simulink model "GuiamentoControle"  (R2024a)
settings: Solver=FixedStepAuto  StartTime=0.0  StopTime=C.Tfim  FixedStep=0.01  MaxStep=0.001  RelTol=1e-3
values from neighbouring files (symbols this model uses):
  C = CondLanc6DOF    [RunGuiamentoDiag.m]    (also in RunGuiamentoFull.m; RunGuiamentoPlots.m; VooUnico6DOF.m)
  cte_grav = 9.8    [CondLanc6DOF.m]    (also in DadosControle.m; DadosMissil.m; Envelope6DOF.m; RunGuiamentoDiag.m)
  D = DadosControle(D)    [Envelope6DOF.m]    (also in ProjContAlt.m = DadosCGInercia(D); ProjRLocus.m = DadosCGInercia(D); RunGuiamentoDiag.m; RunGuiamentoFull.m)
  R2D = 180/pi    (= 57.2957795131)    [DadosControle.m]    (also in Envelope6DOF.m; RunGuiamentoDiag.m; RunGuiamentoFull.m; RunGuiamentoPlots.m)
  T_acel_k_ext = [0.103333333333 0.121666666667 0.126666666667 0.116666666667 0.143333333333 0.196666666667 0.103333333333 0.121666666667 0.126666666667 0.116666666667 0.143333333333 0.193333333333 ... (36 elements, 6x2x3)]    [autopiloto.mat]    (also in autopiloto_antiship.mat = [0.00333333333333 0.00333333333333 0.00333333333333 0.006666)
  T_acel_k_int = [0.788 0.796 0.789 0.757 0.742 0.695 0.792 0.8 0.793 0.761 0.746 0.699 ... (36 elements, 6x2x3)]    [autopiloto.mat]    (also in autopiloto_antiship.mat = [0.786666666667 1.01333333333 1.14666666667 1.18666666667 1.)
  T_at_k_ext = zeros(length(x_CG),length(altitude),length(Mach))    [ProjRLocus.m]    (also in autopiloto.mat = [5.525 6.1 7.1625 8.4375 9.9 12.1875 5.4875 6.0625 7.1125 8.; autopiloto_antiship.mat = [9.33333333333 13.3333333333 18.6666666667 24 34.6666666667 )
  T_at_k_int = zeros(length(x_CG),length(altitude),length(Mach))    [ProjRLocus.m]    (also in autopiloto.mat = [0.788 0.796 0.789 0.757 0.742 0.695 0.792 0.8 0.793 0.761 0; autopiloto_antiship.mat = [0.786666666667 1.01333333333 1.14666666667 1.18666666667 1.)
  vet_altitude = altitude    [ProjRLocus.m]    (also in autopiloto.mat = [10 100]; autopiloto_antiship.mat = [10 100])
  vet_Mach = Mach    [ProjRLocus.m]    (also in autopiloto.mat = [0.6 0.75 0.9]; autopiloto_antiship.mat = [0.6 0.75 0.9 1])
  vet_x_CG = x_CG    [ProjRLocus.m]    (also in autopiloto.mat = [-2.56109748385 -2.4846531203 -2.35211691443 -2.20935548439 ; autopiloto_antiship.mat = [-2.98430726841 -2.86504003942 -2.66873079492 -2.47886843287)
undefined symbols (not defined in the file or in its folder): dados, M_CD, M_CM, M_CMQ, M_CN, Newton, Raphson
libraries: simulink x14, aerolibasang x9, shared6dof x5, sharedutil x3, aerolibatmos2 x1, dspmtrx3 x1
(part 1 of 2)
settings Model: Creator=carlberto-old  LastModifiedBy=mathe
settings SolverCC: AlgebraicLoopSolver=LineSearch
settings DataIOCC: ReturnWorkspaceOutputs=off
settings DebuggingCC: UnconnectedInputMsg=warning  UnconnectedOutputMsg=warning  UnconnectedLineMsg=warning  ArithmeticOperatorsInVariantConditions=warning
settings ModelReferenceCC: EnableRefExpFcnMdlSchedulingChecks=on
settings SFSimCC: SimUseLocalCustomCode=off  CustomCodeUndefinedFunction=UseInterfaceOnly
settings RTWCC: RTWUseLocalCustomCode=off  GPUComputeCapability=3.5

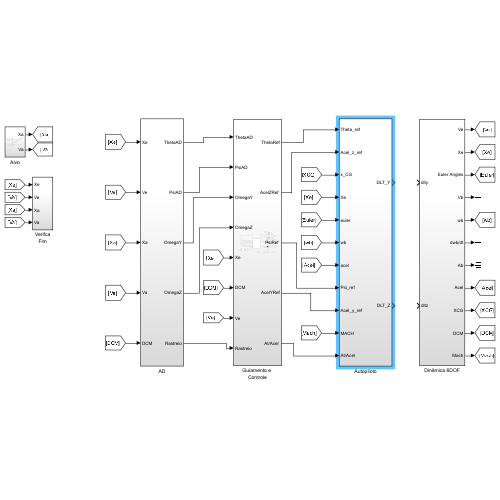
[thumbnail: Simulink's stored preview of the top-level diagram]
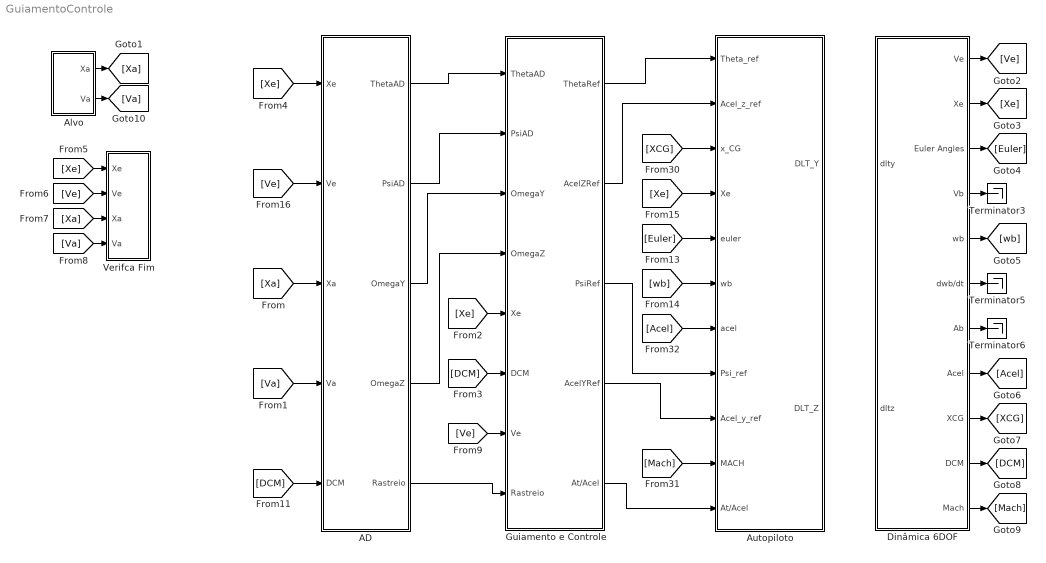
== system GuiamentoControle ==
  "AD " : Subsystem
  Alvo : Subsystem
  Autopiloto : Subsystem
  Dinâmica 6DOF : Subsystem
  Guiamento e Controle : Subsystem
  Terminator3 : Terminator
  Terminator5 : Terminator
  Terminator6 : Terminator
  Verifca Fim : Subsystem
  wires:
  Dinâmica 6DOF/2(Xe) -> [Xe]
  Dinâmica 6DOF/3(Euler Angles) -> [Euler]
  Dinâmica 6DOF/5(wb) -> [wb]
  Dinâmica 6DOF/1(Ve) -> [Ve]
  Dinâmica 6DOF/7(Ab) -> Terminator6/1
  Dinâmica 6DOF/6(dwb/dt) -> Terminator5/1
  Dinâmica 6DOF/4(Vb) -> Terminator3/1
  Dinâmica 6DOF/10(DCM) -> [DCM]
  Dinâmica 6DOF/9(XCG) -> [XCG]
  Dinâmica 6DOF/8(Acel) -> [Acel]
  Dinâmica 6DOF/11(Mach) -> [Mach]
  [XCG] -> Autopiloto/3(x_CG)
  [wb] -> Autopiloto/6(wb)
  [Euler] -> Autopiloto/5(euler)
  [Mach] -> Autopiloto/10(MACH)
  [Acel] -> Autopiloto/7(acel)
  [Xe] -> Autopiloto/4(Xe)
  Guiamento e Controle/5("At/Acel ") -> Autopiloto/11(At/Acel)
  Guiamento e Controle/1(ThetaRef) -> Autopiloto/1(Theta_ref)
  Guiamento e Controle/3("PsiRef ") -> Autopiloto/8(Psi_ref)
  [Xe] -> Guiamento e Controle/5(Xe)
  "AD "/5(Rastreio) -> Guiamento e Controle/8(Rastreio)
  [DCM] -> "AD "/5(DCM)
  [Xe] -> "AD "/1(Xe)
  [Ve] -> "AD "/2(Ve)
  "AD "/1(ThetaAD) -> Guiamento e Controle/1(ThetaAD)
  "AD "/2(PsiAD) -> Guiamento e Controle/2(PsiAD)
  "AD "/3(OmegaY) -> Guiamento e Controle/3(OmegaY)
  "AD "/4(OmegaZ) -> Guiamento e Controle/4(OmegaZ)
  [DCM] -> Guiamento e Controle/6(DCM)
  Alvo/1(Xa) -> [Xa]
  [Xa] -> "AD "/3(Xa)
  Alvo/2(Va) -> [Va]
  [Va] -> "AD "/4(Va)
  [Xe] -> Verifca Fim/1(Xe)
  [Ve] -> Verifca Fim/2(Ve)
  [Xa] -> Verifca Fim/3(Xa)
  [Va] -> Verifca Fim/4(Va)
  Guiamento e Controle/2("AcelZRef ") -> Autopiloto/2(Acel_z_ref)
  Guiamento e Controle/4(AcelYRef) -> Autopiloto/9(Acel_y_ref)
  [Ve] -> Guiamento e Controle/7(Ve)

== system GuiamentoControle/AD  ==
  Xe : Inport
  Ve : Inport  Port=2
  Xa : Inport  Port=3
  Va : Inport  Port=4
  DCM : Inport  Port=5
  AD Ideal : Subsystem
  Subtract1 : Sum  Inputs=+-
  Subtract3 : Sum  Inputs=+-
  ThetaAD : Outport  VectorParamsAs1DForOutWhenUnconnected=off
  PsiAD : Outport  Port=2  VectorParamsAs1DForOutWhenUnconnected=off
  OmegaY : Outport  Port=3  VectorParamsAs1DForOutWhenUnconnected=off
  OmegaZ : Outport  Port=4  VectorParamsAs1DForOutWhenUnconnected=off
  Rastreio : Outport  Port=5  VectorParamsAs1DForOutWhenUnconnected=off
  wires:
  Xa/1 -> Subtract1/1
  Xe/1 -> Subtract1/2
  Va/1 -> Subtract3/1
  Ve/1 -> Subtract3/2
  Subtract1/1 -> AD Ideal/1(Rtm)
  DCM/1 -> AD Ideal/2(DCM)
  Subtract3/1 -> AD Ideal/3(Vtm)
  AD Ideal/1(ThetaAD) -> ThetaAD/1
  AD Ideal/2(PsiAD) -> PsiAD/1
  AD Ideal/3(OmegaY) -> OmegaY/1
  AD Ideal/4(OmegaZ) -> OmegaZ/1
  AD Ideal/5(Rastreio) -> Rastreio/1

== system GuiamentoControle/Alvo ==
  Add : Sum
  Clock : Clock
  Constant : Constant  Value=C.Vxa0
  Constant1 : Constant  Value=C.Vya0
  Constant2 : Constant  Value=C.Vza0
  Constant3 : Constant  Value=C.Xa0
  Constant4 : Constant  Value=C.Ya0
  Constant5 : Constant  Value=-C.Za0
  Divide : Product  Inputs=**
  Mux : Mux  Inputs=3
  Mux1 : Mux  Inputs=3
  To Workspace : ToWorkspace  VariableName=Xa  SaveFormat=Timeseries  SampleTime=-1
  Xa : Outport  VectorParamsAs1DForOutWhenUnconnected=off
  Va : Outport  Port=2  VectorParamsAs1DForOutWhenUnconnected=off
  wires:
  Mux/1 -> Divide/2, Va/1
  Constant/1 -> Mux/1
  Constant1/1 -> Mux/2
  Constant2/1 -> Mux/3
  Constant3/1 -> Mux1/1
  Constant5/1 -> Mux1/3
  Constant4/1 -> Mux1/2
  Clock/1 -> Divide/1
  Divide/1 -> Add/2
  Mux1/1 -> Add/1
  Add/1 -> To Workspace/1, Xa/1

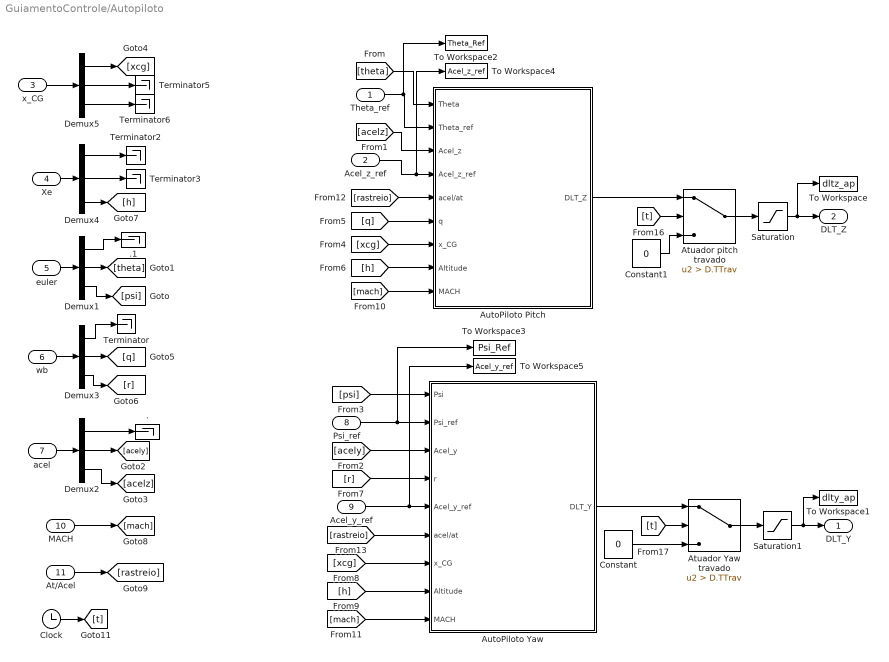
== system GuiamentoControle/Autopiloto ==
  Theta_ref : Inport
  Acel_z_ref : Inport  Port=2
  x_CG : Inport  Port=3
  Xe : Inport  Port=4
  euler : Inport  Port=5
  wb : Inport  Port=6
  acel : Inport  Port=7
  Psi_ref : Inport  Port=8
  Acel_y_ref : Inport  Port=9
  MACH : Inport  Port=10
  At/Acel : Inport  Port=11
  . : Terminator
  .1 : Terminator
  Atuador Yaw travado : Switch  Criteria=u2 > Threshold  Threshold=D.TTrav  SaturateOnIntegerOverflow=off  InputSameDT=off
  Atuador pitch travado : Switch  Criteria=u2 > Threshold  Threshold=D.TTrav  SaturateOnIntegerOverflow=off  InputSameDT=off
  AutoPiloto Pitch : Subsystem
  AutoPiloto Yaw : Subsystem
  Clock : Clock
  Constant : Constant  Value=0
  Constant1 : Constant  Value=0
  Demux{1..5} (5 alike) : Demux  Outputs=3
  Saturation : Saturate  UpperLimit=D.Dlt_max  LowerLimit=-D.Dlt_max
  Saturation1 : Saturate  UpperLimit=D.Dlt_max  LowerLimit=-D.Dlt_max
  Terminator{,2..3,5..6} (5 alike) : Terminator
  To Workspace : ToWorkspace  VariableName=dltz_ap  SaveFormat=Timeseries  SampleTime=-1
  To Workspace1 : ToWorkspace  VariableName=dlty_ap  SaveFormat=Timeseries  SampleTime=-1
  To Workspace2 : ToWorkspace  VariableName=Theta_Ref  SaveFormat=Timeseries  SampleTime=-1
  To Workspace3 : ToWorkspace  VariableName=Psi_Ref  SaveFormat=Timeseries  SampleTime=-1
  To Workspace4 : ToWorkspace  VariableName=Acel_z_ref  SaveFormat=Timeseries  SampleTime=-1
  To Workspace5 : ToWorkspace  VariableName=Acel_y_ref  SaveFormat=Timeseries  SampleTime=-1
  DLT_Y : Outport  VectorParamsAs1DForOutWhenUnconnected=off
  DLT_Z : Outport  Port=2  VectorParamsAs1DForOutWhenUnconnected=off
  wires:
  Theta_ref/1 -> To Workspace2/1, AutoPiloto Pitch/2(Theta_ref)
  acel/1 -> Demux2/1
  wb/1 -> Demux3/1
  Xe/1 -> Demux4/1
  euler/1 -> Demux1/1
  Demux2/1 -> ./1
  Demux4/1 -> Terminator2/1
  Demux4/2 -> Terminator3/1
  Demux3/1 -> Terminator/1
  Psi_ref/1 -> To Workspace3/1, AutoPiloto Yaw/2(Psi_ref)
  Acel_y_ref/1 -> To Workspace5/1, AutoPiloto Yaw/5(Acel_y_ref)
  Acel_z_ref/1 -> To Workspace4/1, AutoPiloto Pitch/4(Acel_z_ref)
  Demux1/1 -> .1/1
  x_CG/1 -> Demux5/1
  Demux5/2 -> Terminator5/1
  Demux5/3 -> Terminator6/1
  Constant/1 -> Atuador Yaw travado/3
  Demux1/2 -> [theta]
  Demux1/3 -> [psi]
  [theta] -> AutoPiloto Pitch/1(Theta)
  Demux2/3 -> [acelz]
  Demux2/2 -> [acely]
  [acely] -> AutoPiloto Yaw/3(Acel_y)
  [psi] -> AutoPiloto Yaw/1(Psi)
  Demux5/1 -> [xcg]
  [xcg] -> AutoPiloto Pitch/7(x_CG)
  Demux3/2 -> [q]
  Demux3/3 -> [r]
  [q] -> AutoPiloto Pitch/6(q)
  Demux4/3 -> [h]
  [h] -> AutoPiloto Pitch/8(Altitude)
  [r] -> AutoPiloto Yaw/4(r)
  [xcg] -> AutoPiloto Yaw/7(x_CG)
  [h] -> AutoPiloto Yaw/8(Altitude)
  MACH/1 -> [mach]
  [mach] -> AutoPiloto Pitch/9(MACH)
  [mach] -> AutoPiloto Yaw/9(MACH)
  At/Acel/1 -> [rastreio]
  [rastreio] -> AutoPiloto Pitch/5(acel/at)
  [rastreio] -> AutoPiloto Yaw/6(acel/at)
  Constant1/1 -> Atuador pitch travado/3
  Atuador pitch travado/1 -> Saturation/1
  Saturation/1 -> To Workspace/1, DLT_Z/1
  Atuador Yaw travado/1 -> Saturation1/1
  Saturation1/1 -> DLT_Y/1, To Workspace1/1
  Clock/1 -> [t]
  [t] -> Atuador pitch travado/2
  [t] -> Atuador Yaw travado/2
  [acelz] -> AutoPiloto Pitch/3(Acel_z)
  AutoPiloto Pitch/1(DLT_Z) -> Atuador pitch travado/1
  AutoPiloto Yaw/1(DLT_Y) -> Atuador Yaw travado/1

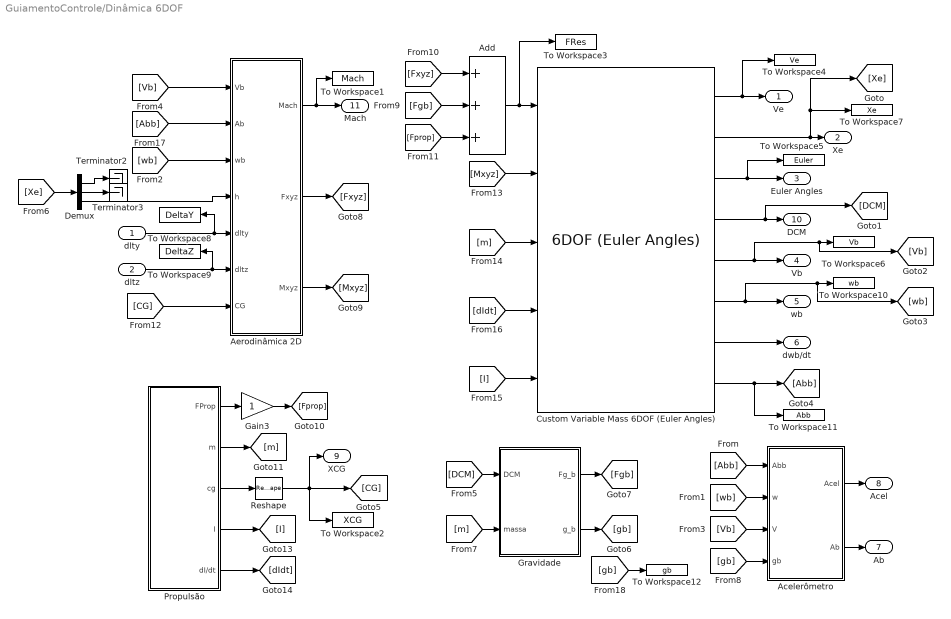
== system GuiamentoControle/Dinâmica 6DOF ==
  dlty : Inport
  dltz : Inport  Port=2
  Acelerômetro : Subsystem
  Add : Sum  Inputs=+++
  Aerodinâmica 2D : Subsystem
  Custom Variable Mass 6DOF (Euler Angles) : shared6dof/6DOF (Euler Angles)  units=Metric (MKS)  mtype=Custom Variable  rep=Euler Angles  xme_0=[C.Xm0 C.Ym0 -C.Zm0]  Vm_0="[C.Vmx0  C.Vmy0   C.Vmz0]"  eul_0="[C.Phim0  C.Tetam0   C.Psim0]"  pm_0=[C.p0 C.q0 C.r0]  mass_0=1.0  mass_e=0.5  mass_f=2.0  inertia=eye(3)  inertia_e=eye(3)  inertia_f=2*eye(3)  k_quat=1.0  vre_flag=off  abi_flag=off  aMode=aMode  xme_statename=''  Vm_statename=''  eul_statename=''  quat_statename=''  pm_statename=''  mass_statename=''
  Demux : Demux  Outputs=3
  Gain3 : Gain
  Gravidade : Subsystem
  Propulsão : Subsystem
  Reshape : Reshape
  Terminator2 : Terminator
  Terminator3 : Terminator
  To Workspace1 : ToWorkspace  VariableName=Mach  SaveFormat=Timeseries  SampleTime=-1
  To Workspace10 : ToWorkspace  VariableName=wb  SaveFormat=Timeseries  SampleTime=-1
  To Workspace11 : ToWorkspace  VariableName=Abb  SaveFormat=Timeseries  SampleTime=-1
  To Workspace12 : ToWorkspace  VariableName=gb  SaveFormat=Timeseries  SampleTime=-1
  To Workspace2 : ToWorkspace  VariableName=XCG  SaveFormat=Timeseries  SampleTime=-1
  To Workspace3 : ToWorkspace  VariableName=FRes  SaveFormat=Timeseries  SampleTime=-1
  To Workspace4 : ToWorkspace  VariableName=Ve  SaveFormat=Timeseries  SampleTime=-1
  To Workspace5 : ToWorkspace  VariableName=Euler  SaveFormat=Timeseries  SampleTime=-1
  To Workspace6 : ToWorkspace  VariableName=Vb  SaveFormat=Timeseries  SampleTime=-1
  To Workspace7 : ToWorkspace  VariableName=Xe  SaveFormat=Timeseries  SampleTime=-1
  To Workspace8 : ToWorkspace  VariableName=DeltaY  SaveFormat=Timeseries  SampleTime=-1
  To Workspace9 : ToWorkspace  VariableName=DeltaZ  SaveFormat=Timeseries  SampleTime=-1
  Ve : Outport  VectorParamsAs1DForOutWhenUnconnected=off
  Xe : Outport  Port=2  VectorParamsAs1DForOutWhenUnconnected=off
  Euler Angles : Outport  Port=3  VectorParamsAs1DForOutWhenUnconnected=off
  Vb : Outport  Port=4  VectorParamsAs1DForOutWhenUnconnected=off
  wb : Outport  Port=5  VectorParamsAs1DForOutWhenUnconnected=off
  dwb/dt : Outport  Port=6  VectorParamsAs1DForOutWhenUnconnected=off
  Ab : Outport  Port=7  VectorParamsAs1DForOutWhenUnconnected=off
  Acel : Outport  Port=8  VectorParamsAs1DForOutWhenUnconnected=off
  XCG : Outport  Port=9  VectorParamsAs1DForOutWhenUnconnected=off
  DCM : Outport  Port=10  VectorParamsAs1DForOutWhenUnconnected=off
  Mach : Outport  Port=11  VectorParamsAs1DForOutWhenUnconnected=off
  wires:
  Custom Variable Mass 6DOF (Euler Angles)/1 -> To Workspace4/1, Ve/1
  Custom Variable Mass 6DOF (Euler Angles)/3 -> To Workspace5/1, Euler Angles/1
  Custom Variable Mass 6DOF (Euler Angles)/7 -> dwb/dt/1
  Add/1 -> To Workspace3/1, Custom Variable Mass 6DOF (Euler Angles)/1
  Custom Variable Mass 6DOF (Euler Angles)/4 -> DCM/1, [DCM]
  Reshape/1 -> XCG/1, [CG], To Workspace2/1
  Propulsão/3(cg) -> Reshape/1
  [Abb] -> Acelerômetro/1(Abb)
  [wb] -> Acelerômetro/2(w)
  [Vb] -> Acelerômetro/3(V)
  [DCM] -> Gravidade/1(DCM)
  Acelerômetro/2(Ab) -> Ab/1
  [gb] -> Acelerômetro/4(gb)
  Propulsão/2(m) -> [m]
  Propulsão/4(I) -> [I]
  Propulsão/5(dI/dt) -> [dIdt]
  [m] -> Custom Variable Mass 6DOF (Euler Angles)/3
  [I] -> Custom Variable Mass 6DOF (Euler Angles)/5
  [dIdt] -> Custom Variable Mass 6DOF (Euler Angles)/4
  Custom Variable Mass 6DOF (Euler Angles)/6 -> [wb], To Workspace10/1, wb/1
  Custom Variable Mass 6DOF (Euler Angles)/8 -> [Abb], To Workspace11/1
  Custom Variable Mass 6DOF (Euler Angles)/5 -> To Workspace6/1, [Vb], Vb/1
  [m] -> Gravidade/2(massa)
  [Fxyz] -> Add/1
  Gravidade/1(Fg_b) -> [Fgb]
  [Mxyz] -> Custom Variable Mass 6DOF (Euler Angles)/2
  Acelerômetro/1(Acel) -> Acel/1
  Gravidade/2(g_b) -> [gb]
  [Fgb] -> Add/2
  [Fprop] -> Add/3
  Demux/1 -> Terminator2/1
  [Xe] -> Demux/1
  [CG] -> Aerodinâmica 2D/7(CG)
  dlty/1 -> To Workspace8/1, Aerodinâmica 2D/5(dlty)
  Demux/2 -> Terminator3/1
  Aerodinâmica 2D/1(Mach) -> To Workspace1/1, Mach/1
  Aerodinâmica 2D/3(Mxyz) -> [Mxyz]
  [wb] -> Aerodinâmica 2D/3(wb)
  [Vb] -> Aerodinâmica 2D/1(Vb)
  [Abb] -> Aerodinâmica 2D/2(Ab)
  Aerodinâmica 2D/2(Fxyz) -> [Fxyz]
  Demux/3 -> Aerodinâmica 2D/4(h)
  dltz/1 -> Aerodinâmica 2D/6(dltz), To Workspace9/1
  Propulsão/1(FProp) -> Gain3/1
  Gain3/1 -> [Fprop]
  Custom Variable Mass 6DOF (Euler Angles)/2 -> [Xe], To Workspace7/1, Xe/1
  [gb] -> To Workspace12/1

== system GuiamentoControle/Guiamento e Controle ==
  ThetaAD : Inport
  PsiAD : Inport  Port=2
  OmegaY : Inport  Port=3
  OmegaZ : Inport  Port=4
  Xe : Inport  Port=5
  DCM : Inport  Port=6
  Ve : Inport  Port=7
  Rastreio : Inport  Port=8
   {,1..3} (4 alike) : Switch  Criteria=u2 > Threshold  SaturateOnIntegerOverflow=off  InputSameDT=off
  Clock : Clock
  Compare To Constant : simulink/Logic and Bit Operations/Compare To Constant  relop=>=  const=C.TLaser  OutDataTypeStr=boolean  ZeroCross=off
  Constant1 : Constant  Value=0
  Constant2 : Constant  Value=0
  Controle de Atitude : Subsystem
  Guiamento Terminal : Subsystem
  Sqrt : Sqrt
  Terminator : Terminator
  dot : aerolibasang/Incidence, Sideslip, & Airspeed/dot  SystemSampleTime=-1  VariantActivationTime=update diagram  AllowFlexibleInterface=on  Latency=0  AutoFrameSizeCalculation=off
  ThetaRef : Outport  VectorParamsAs1DForOutWhenUnconnected=off
  "AcelZRef " : Outport  Port=2  VectorParamsAs1DForOutWhenUnconnected=off
  "PsiRef " : Outport  Port=3  VectorParamsAs1DForOutWhenUnconnected=off
  AcelYRef : Outport  Port=4  VectorParamsAs1DForOutWhenUnconnected=off
  "At/Acel " : Outport  Port=5  VectorParamsAs1DForOutWhenUnconnected=off
  wires:
  Xe/1 -> Controle de Atitude/1(Xe)
  Rastreio/1 -> Guiamento Terminal/6(Rastreio)
  Constant2/1 -> " 1"/1, " "/1
  " "/1 -> "PsiRef "/1
  Controle de Atitude/1(psiREF) -> " "/3
  Controle de Atitude/2(ThetaRef) -> ThetaRef/1, " 1"/3
  " 2"/1 -> "AcelZRef "/1
  " 3"/1 -> AcelYRef/1
  Constant1/1 -> " 2"/3, " 3"/3
  OmegaY/1 -> Guiamento Terminal/2(OmegaY)
  OmegaZ/1 -> Guiamento Terminal/4(OmegaZ)
  PsiAD/1 -> Guiamento Terminal/3(PsiAD)
  ThetaAD/1 -> Guiamento Terminal/1(TetaAD)
  DCM/1 -> Guiamento Terminal/5(DCM)
  Guiamento Terminal/1(AcelZCom) -> " 2"/1
  Guiamento Terminal/2(AcelYCom) -> " 3"/1
  Clock/1 -> Compare To Constant/1
  Compare To Constant/1 -> " "/2, " 1"/2, " 2"/2, " 3"/2, "At/Acel "/1
  Sqrt/1 -> Guiamento Terminal/7(|Vm|)
  Ve/1 -> dot/1
  dot/1 -> Sqrt/1
  " 1"/1 -> Terminator/1

== system GuiamentoControle/Verifca Fim ==
  Xe : Inport
  Ve : Inport  Port=2
  Xa : Inport  Port=3
  Va : Inport  Port=4
  Bingo : Subsystem
  Clock : Clock
  Impacto com solo : Subsystem
  Parada: Fuga do alvo : Subsystem
  Parada: V < VMin : Subsystem
  Subtract1 : Sum  Inputs=-+
  Subtract3 : Sum  Inputs=-+
  wires:
  Xe/1 -> Impacto com solo/1(Rtm), Subtract3/1
  Xa/1 -> Subtract3/2
  Subtract3/1 -> Bingo/1(Rtm), Parada: Fuga do alvo/1(Rtm)
  Ve/1 -> Parada: V < VMin/1(V), Subtract1/1
  Clock/1 -> Parada: V < VMin/2(t), Parada: Fuga do alvo/3(t)
  Subtract1/1 -> Parada: Fuga do alvo/2(Vtm)
  Va/1 -> Subtract1/2

== system GuiamentoControle/AD /AD Ideal ==
  Rtm : Inport
  DCM : Inport  Port=2
  Vtm : Inport  Port=3
  3x3 Cross Product : sharedutil/3x3 Cross Product  aMode=aMode
  Atan1 : Trigonometry  Operator=atan2
  Atan2 : Trigonometry  Operator=atan2
  Demux1 : Demux  Outputs=3
  Demux3 : Demux  Outputs=3
  Divide1 : Product  Inputs=*/
  Gain1 : Gain  Gain=-1
  Gain4 : Gain
  "Limites de Rastreio " : Subsystem
  "Si->Sb " : shared6dof/6DOF (Euler Angles)/transform to Inertial axes   SystemSampleTime=-1
      settings: SourceProductName=Aerospace Blockset
  Si->Sb1 : shared6dof/6DOF (Euler Angles)/transform to Inertial axes   SystemSampleTime=-1
      settings: SourceProductName=Aerospace Blockset
  Terminator3 : Terminator
  dot : aerolibasang/Incidence, Sideslip, & Airspeed/dot  SystemSampleTime=-1
      settings: SourceProductName=Aerospace Blockset
  ThetaAD : Outport  VectorParamsAs1DForOutWhenUnconnected=off
  PsiAD : Outport  Port=2  VectorParamsAs1DForOutWhenUnconnected=off
  OmegaY : Outport  Port=3  VectorParamsAs1DForOutWhenUnconnected=off
  OmegaZ : Outport  Port=4  VectorParamsAs1DForOutWhenUnconnected=off
  Rastreio : Outport  Port=5  VectorParamsAs1DForOutWhenUnconnected=off
  wires:
  Divide1/1 -> Demux3/1
  Atan1/1 -> Gain1/1
  Vtm/1 -> "Si->Sb "/1
  Demux1/3 -> Atan1/1
  Gain1/1 -> "Limites de Rastreio "/1(ThetaAD)
  Rtm/1 -> Si->Sb1/1
  "Limites de Rastreio "/2("PsiAD ") -> PsiAD/1
  Demux1/2 -> Atan2/1
  Demux3/1 -> Terminator3/1
  Demux3/3 -> "Limites de Rastreio "/4(OmegaZ)
  "Limites de Rastreio "/5(Rastreio) -> Rastreio/1
  Gain4/1 -> "Limites de Rastreio "/2(PsiAD)
  "Si->Sb "/1 -> 3x3 Cross Product/2
  3x3 Cross Product/1 -> Divide1/1
  "Limites de Rastreio "/1("ThetaAD ") -> ThetaAD/1
  "Limites de Rastreio "/3("OmegaY ") -> OmegaY/1
  DCM/1 -> "Si->Sb "/2, Si->Sb1/2
  Si->Sb1/1 -> 3x3 Cross Product/1, "Limites de Rastreio "/5(RTM), dot/1, Demux1/1
  "Limites de Rastreio "/4("OmegaZ ") -> OmegaZ/1
  Atan2/1 -> Gain4/1
  dot/1 -> Divide1/2
  Demux3/2 -> "Limites de Rastreio "/3(OmegaY)
  Demux1/1 -> Atan1/2, Atan2/2

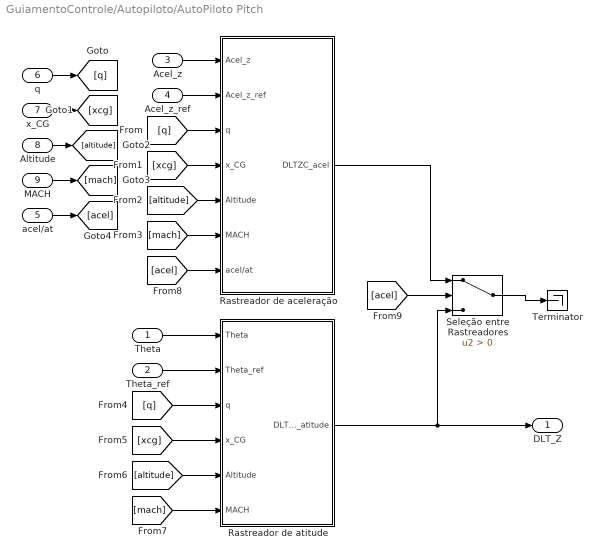
== system GuiamentoControle/Autopiloto/AutoPiloto Pitch ==
  Theta : Inport
  Theta_ref : Inport  Port=2
  Acel_z : Inport  Port=3
  Acel_z_ref : Inport  Port=4
  acel/at : Inport  Port=5
  q : Inport  Port=6
  x_CG : Inport  Port=7
  Altitude : Inport  Port=8
  MACH : Inport  Port=9
  Rastreador de aceleração : Subsystem
  Rastreador de atitude : Subsystem
  Seleção entre Rastreadores : Switch  Criteria=u2 > Threshold  SaturateOnIntegerOverflow=off  InputSameDT=off
  Terminator : Terminator
  DLT_Z : Outport  VectorParamsAs1DForOutWhenUnconnected=off
  wires:
  Theta/1 -> Rastreador de atitude/1(Theta)
  Theta_ref/1 -> Rastreador de atitude/2(Theta_ref)
  Acel_z/1 -> Rastreador de aceleração/1(Acel_z)
  Acel_z_ref/1 -> Rastreador de aceleração/2(Acel_z_ref)
  acel/at/1 -> [acel]
  [q] -> Rastreador de aceleração/3(q)
  [xcg] -> Rastreador de aceleração/4(x_CG)
  [altitude] -> Rastreador de aceleração/5(Altitude)
  [mach] -> Rastreador de aceleração/6(MACH)
  [q] -> Rastreador de atitude/3(q)
  [xcg] -> Rastreador de atitude/4(x_CG)
  [altitude] -> Rastreador de atitude/5(Altitude)
  [mach] -> Rastreador de atitude/6(MACH)
  x_CG/1 -> [xcg]
  q/1 -> [q]
  MACH/1 -> [mach]
  Altitude/1 -> [altitude]
  Rastreador de atitude/1(DLTZC_atitude) -> DLT_Z/1, Seleção entre Rastreadores/3
  [acel] -> Rastreador de aceleração/7(acel/at)
  [acel] -> Seleção entre Rastreadores/2
  Rastreador de aceleração/1(DLTZC_acel) -> Seleção entre Rastreadores/1
  Seleção entre Rastreadores/1 -> Terminator/1

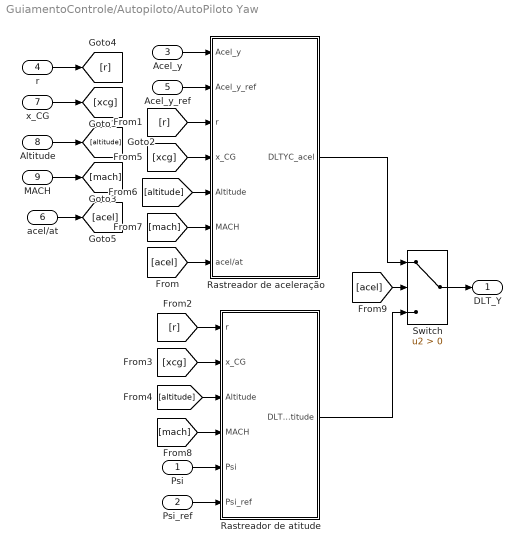
== system GuiamentoControle/Autopiloto/AutoPiloto Yaw ==
  Psi : Inport
  Psi_ref : Inport  Port=2
  Acel_y : Inport  Port=3
  r : Inport  Port=4
  Acel_y_ref : Inport  Port=5
  acel/at : Inport  Port=6
  x_CG : Inport  Port=7
  Altitude : Inport  Port=8
  MACH : Inport  Port=9
  Rastreador de aceleração : Subsystem
  Rastreador de atitude : Subsystem
  Switch : Switch  Criteria=u2 > Threshold  SaturateOnIntegerOverflow=off  InputSameDT=off
  DLT_Y : Outport  VectorParamsAs1DForOutWhenUnconnected=off
  wires:
  Switch/1 -> DLT_Y/1
  Psi/1 -> Rastreador de atitude/5(Psi)
  Rastreador de atitude/1(DLTYC_atitude) -> Switch/3
  Acel_y/1 -> Rastreador de aceleração/1(Acel_y)
  Acel_y_ref/1 -> Rastreador de aceleração/2(Acel_y_ref)
  Rastreador de aceleração/1(DLTYC_acel) -> Switch/1
  acel/at/1 -> [acel]
  r/1 -> [r]
  x_CG/1 -> [xcg]
  Altitude/1 -> [altitude]
  MACH/1 -> [mach]
  [r] -> Rastreador de aceleração/3(r)
  [xcg] -> Rastreador de aceleração/4(x_CG)
  [altitude] -> Rastreador de aceleração/5(Altitude)
  [mach] -> Rastreador de aceleração/6(MACH)
  [r] -> Rastreador de atitude/1(r)
  [xcg] -> Rastreador de atitude/2(x_CG)
  [altitude] -> Rastreador de atitude/3(Altitude)
  [mach] -> Rastreador de atitude/4(MACH)
  [acel] -> Rastreador de aceleração/7(acel/at)
  [acel] -> Switch/2
  Psi_ref/1 -> Rastreador de atitude/6(Psi_ref)

== system GuiamentoControle/Dinâmica 6DOF/Acelerômetro ==
  Abb : Inport
  w : Inport  Port=2
  V : Inport  Port=3
  gb : Inport  Port=4
  Add1 : Sum
  Add2 : Sum  Inputs=+-
  To Workspace4 : ToWorkspace  VariableName=Acel  SaveFormat=Timeseries  SampleTime=-1
  To Workspace5 : ToWorkspace  VariableName=Ab  SaveFormat=Timeseries  SampleTime=-1
  w x V : sharedutil/3x3 Cross Product  aMode=aMode
  Acel : Outport  VectorParamsAs1DForOutWhenUnconnected=off
  Ab : Outport  Port=2  VectorParamsAs1DForOutWhenUnconnected=off
  wires:
  V/1 -> w x V/2
  w/1 -> w x V/1
  Add1/1 -> Add2/1, Ab/1, To Workspace5/1
  Add2/1 -> To Workspace4/1, Acel/1
  gb/1 -> Add2/2
  w x V/1 -> Add1/2
  Abb/1 -> Add1/1

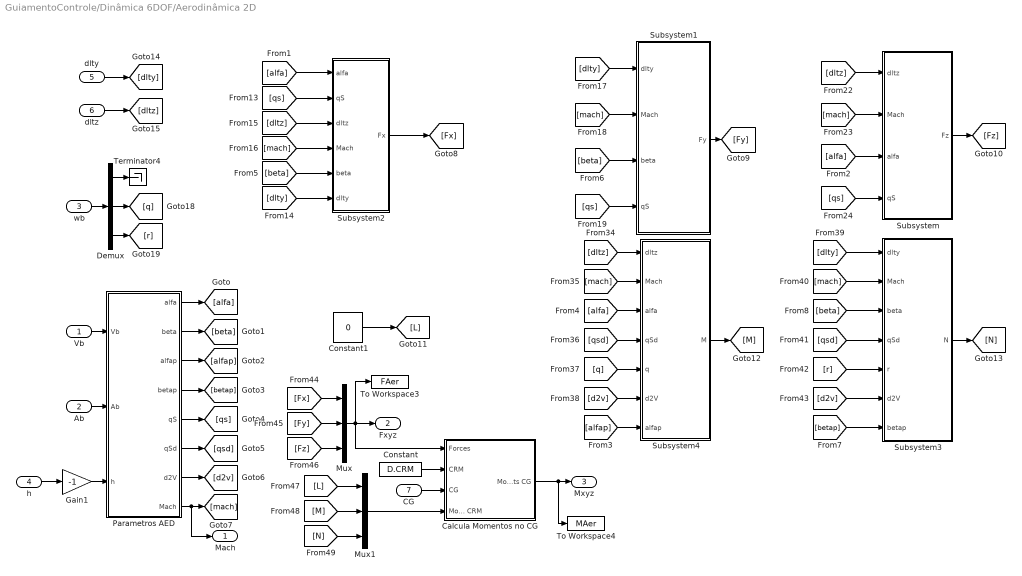
== system GuiamentoControle/Dinâmica 6DOF/Aerodinâmica 2D ==
  Vb : Inport
  Ab : Inport  Port=2
  wb : Inport  Port=3
  h : Inport  Port=4
  dlty : Inport  Port=5
  dltz : Inport  Port=6
  CG : Inport  Port=7
  Calcula Momentos no CG : Subsystem
  Constant : Constant  Value=D.CRM
  Constant1 : Constant  Value=0
  Demux : Demux  Outputs=3
  Gain1 : Gain  Gain=-1
  Mux : Mux  Inputs=3
  Mux1 : Mux  Inputs=3
  Parametros AED : Subsystem
  Subsystem : Subsystem
  Subsystem1 : Subsystem
  Subsystem2 : Subsystem
  Subsystem3 : Subsystem
  Subsystem4 : Subsystem
  Terminator4 : Terminator
  To Workspace3 : ToWorkspace  VariableName=FAer  SaveFormat=Timeseries  SampleTime=-1
  To Workspace4 : ToWorkspace  VariableName=MAer  SaveFormat=Timeseries  SampleTime=-1
  Mach : Outport  VectorParamsAs1DForOutWhenUnconnected=off
  Fxyz : Outport  Port=2  VectorParamsAs1DForOutWhenUnconnected=off
  Mxyz : Outport  Port=3  VectorParamsAs1DForOutWhenUnconnected=off
  wires:
  Mux1/1 -> Calcula Momentos no CG/4(Moments CRM)
  wb/1 -> Demux/1
  Vb/1 -> Parametros AED/1(Vb)
  Ab/1 -> Parametros AED/2(Ab)
  CG/1 -> Calcula Momentos no CG/3(CG)
  Constant/1 -> Calcula Momentos no CG/2(CRM)
  Calcula Momentos no CG/1(Moments CG) -> To Workspace4/1, Mxyz/1
  Parametros AED/1(alfa) -> [alfa]
  [alfa] -> Subsystem2/1(alfa)
  [alfa] -> Subsystem/3(alfa)
  [alfa] -> Subsystem4/3(alfa)
  Parametros AED/2(beta) -> [beta]
  [beta] -> Subsystem1/3(beta)
  [beta] -> Subsystem3/3(beta)
  Parametros AED/3(alfap) -> [alfap]
  Parametros AED/4(betap) -> [betap]
  Parametros AED/5(qS) -> [qs]
  Parametros AED/6(qSd) -> [qsd]
  Parametros AED/7(d2V) -> [d2v]
  Parametros AED/8(Mach) -> Mach/1, [mach]
  [qs] -> Subsystem2/2(qS)
  [dlty] -> Subsystem2/6(dlty)
  [dltz] -> Subsystem2/3(dltz)
  [mach] -> Subsystem2/4("Mach ")
  [dlty] -> Subsystem1/1("dlty ")
  [mach] -> Subsystem1/2(Mach)
  [qs] -> Subsystem1/4(qS)
  Subsystem1/1(Fy) -> [Fy]
  [dltz] -> Subsystem/1(dltz)
  [mach] -> Subsystem/2("Mach ")
  [qs] -> Subsystem/4(qS)
  Subsystem/1(Fz) -> [Fz]
  [dltz] -> Subsystem4/1(dltz)
  [mach] -> Subsystem4/2(Mach)
  [qsd] -> Subsystem4/4(qSd)
  [q] -> Subsystem4/5(q)
  [d2v] -> Subsystem4/6(d2V)
  Subsystem4/1(M) -> [M]
  [dlty] -> Subsystem3/1(dlty)
  [mach] -> Subsystem3/2(Mach)
  [qsd] -> Subsystem3/4(qSd)
  [r] -> Subsystem3/5(r)
  [d2v] -> Subsystem3/6(d2V)
  Subsystem3/1(N) -> [N]
  [Fx] -> Mux/1
  [Fy] -> Mux/2
  [Fz] -> Mux/3
  [L] -> Mux1/1
  [M] -> Mux1/2
  [N] -> Mux1/3
  dlty/1 -> [dlty]
  dltz/1 -> [dltz]
  Demux/1 -> Terminator4/1
  Demux/2 -> [q]
  Demux/3 -> [r]
  Constant1/1 -> [L]
  [beta] -> Subsystem2/5(beta)
  [alfap] -> Subsystem4/7(alfap)
  [betap] -> Subsystem3/7(betap)
  Subsystem2/1(Fx) -> [Fx]
  Mux/1 -> Calcula Momentos no CG/1(Forces), Fxyz/1, To Workspace3/1
  h/1 -> Gain1/1
  Gain1/1 -> Parametros AED/3(h)

== system GuiamentoControle/Dinâmica 6DOF/Gravidade ==
  DCM : Inport
  massa : Inport  Port=2
  Constant2 : Constant  Value=0
  Constant3 : Constant  Value=0
  Constant4 : Constant  Value=cte_grav
  Mux : Mux  Inputs=3
  Product : Product
  "transform to Inertial axes " : shared6dof/6DOF (Euler Angles)/transform to Inertial axes   SystemSampleTime=-1
      settings: SourceProductName=Aerospace Blockset
  Fg_b : Outport  VectorParamsAs1DForOutWhenUnconnected=off
  g_b : Outport  Port=2  VectorParamsAs1DForOutWhenUnconnected=off
  wires:
  Constant3/1 -> Mux/2
  Constant2/1 -> Mux/1
  Constant4/1 -> Mux/3
  DCM/1 -> "transform to Inertial axes "/2
  massa/1 -> Product/2
  Product/1 -> Fg_b/1
  "transform to Inertial axes "/1 -> g_b/1, Product/1
  Mux/1 -> "transform to Inertial axes "/1

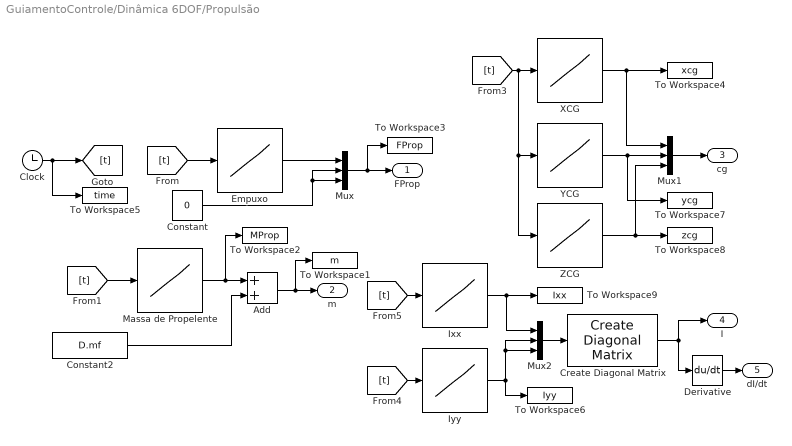
== system GuiamentoControle/Dinâmica 6DOF/Propulsão ==
  Add : Sum
  Clock : Clock
  Constant : Constant  Value=0
  Constant2 : Constant  Value=D.mf
  Create Diagonal Matrix : dspmtrx3/Create Diagonal Matrix
      settings: SourceProductName=DSP System Toolbox
  Derivative : Derivative
  "Empuxo " : Lookup_n-D  NumberOfTableDimensions=1  BreakpointsForDimension1=D.VProp(:,1)  Table=D.VProp(:,2)  ExtrapMethod=Clip  InternalRulePriority=Speed  RndMeth=Simplest
  Ixx : Lookup_n-D  NumberOfTableDimensions=1  BreakpointsForDimension1=D.IMissil(:,1)  Table=D.IMissil(:,2)  ExtrapMethod=Clip  InternalRulePriority=Speed  RndMeth=Simplest
  Iyy : Lookup_n-D  NumberOfTableDimensions=1  BreakpointsForDimension1=D.IMissil(:,1)  Table=D.IMissil(:,3)  ExtrapMethod=Clip  InternalRulePriority=Speed  RndMeth=Simplest
  Massa de Propelente : Lookup_n-D  NumberOfTableDimensions=1  BreakpointsForDimension1=D.VProp(:,1)  Table=D.VProp(:,3)  ExtrapMethod=Clip  InternalRulePriority=Speed  RndMeth=Simplest
  Mux : Mux  Inputs=3
  Mux1 : Mux  Inputs=3
  Mux2 : Mux  Inputs=3
  To Workspace1 : ToWorkspace  VariableName=m  SaveFormat=Timeseries  SampleTime=-1
  To Workspace2 : ToWorkspace  VariableName=MProp  SaveFormat=Timeseries  SampleTime=-1
  To Workspace3 : ToWorkspace  VariableName=FProp  SaveFormat=Timeseries  SampleTime=-1
  To Workspace4 : ToWorkspace  VariableName=xcg  SaveFormat=Timeseries  SampleTime=-1
  To Workspace5 : ToWorkspace  VariableName=time  SaveFormat=Timeseries  SampleTime=-1
  To Workspace6 : ToWorkspace  VariableName=Iyy  SaveFormat=Timeseries  SampleTime=-1
  To Workspace7 : ToWorkspace  VariableName=ycg  SaveFormat=Timeseries  SampleTime=-1
  To Workspace8 : ToWorkspace  VariableName=zcg  SaveFormat=Timeseries  SampleTime=-1
  To Workspace9 : ToWorkspace  VariableName=Ixx  SaveFormat=Timeseries  SampleTime=-1
  "XCG " : Lookup_n-D  NumberOfTableDimensions=1  BreakpointsForDimension1=D.CGMissil(:,1)  Table=D.CGMissil(:,2)  ExtrapMethod=Clip  InternalRulePriority=Speed  RndMeth=Simplest
  "YCG " : Lookup_n-D  NumberOfTableDimensions=1  BreakpointsForDimension1=D.CGMissil(:,1)  Table=D.CGMissil(:,3)  ExtrapMethod=Clip  InternalRulePriority=Speed  RndMeth=Simplest
  "ZCG " : Lookup_n-D  NumberOfTableDimensions=1  BreakpointsForDimension1=D.CGMissil(:,1)  Table=D.CGMissil(:,4)  ExtrapMethod=Clip  InternalRulePriority=Speed  RndMeth=Simplest
  FProp : Outport  VectorParamsAs1DForOutWhenUnconnected=off
  m : Outport  Port=2  VectorParamsAs1DForOutWhenUnconnected=off
  cg : Outport  Port=3  VectorParamsAs1DForOutWhenUnconnected=off
  I : Outport  Port=4  VectorParamsAs1DForOutWhenUnconnected=off
  dI/dt : Outport  Port=5  VectorParamsAs1DForOutWhenUnconnected=off
  wires:
  Mux/1 -> FProp/1, To Workspace3/1
  "Empuxo "/1 -> Mux/1
  Constant/1 -> Mux/3, Mux/2
  Massa de Propelente/1 -> To Workspace2/1, Add/1
  Add/1 -> m/1, To Workspace1/1
  Constant2/1 -> Add/2
  Derivative/1 -> dI/dt/1
  Mux1/1 -> cg/1
  "XCG "/1 -> To Workspace4/1, Mux1/1
  Create Diagonal Matrix/1 -> I/1, Derivative/1
  Ixx/1 -> To Workspace9/1, Mux2/1
  Iyy/1 -> To Workspace6/1, Mux2/3, Mux2/2
  Mux2/1 -> Create Diagonal Matrix/1
  Clock/1 -> [t], To Workspace5/1
  [t] -> "Empuxo "/1
  [t] -> Massa de Propelente/1
  [t] -> "ZCG "/1, "YCG "/1, "XCG "/1
  [t] -> Ixx/1
  [t] -> Iyy/1
  "YCG "/1 -> To Workspace7/1, Mux1/2
  "ZCG "/1 -> Mux1/3, To Workspace8/1

== system GuiamentoControle/Guiamento e Controle/Controle de Atitude ==
  Xe : Inport
  " 1" : Switch  Criteria=u2 > Threshold  Threshold=D.TTrav  SaturateOnIntegerOverflow=off  InputSameDT=off
  " 2" : Switch  Criteria=u2 > Threshold  Threshold=D.TTrav  SaturateOnIntegerOverflow=off  InputSameDT=off
  Clock : Clock
  Constant2 : Constant  Value=0
  Constant3 : Constant  Value=C.AltCruz
  Constant4 : Constant  Value=C.Rumo0
  Demux1 : Demux  Outputs=3
  Gain : Gain  Gain=D.KAlt
  Saturation1 : Saturate  UpperLimit=D.AngSubMax  LowerLimit=-D.AngSubMax
  Sum : Sum  Inputs=|++
  Terminator1 : Terminator
  Terminator4 : Terminator
  To Workspace : ToWorkspace  VariableName=PsiRef  SaveFormat=Timeseries  SampleTime=-1
  To Workspace1 : ToWorkspace  VariableName=ThetaRef  SaveFormat=Timeseries  SampleTime=-1
  psiREF : Outport  VectorParamsAs1DForOutWhenUnconnected=off
  ThetaRef : Outport  Port=2  VectorParamsAs1DForOutWhenUnconnected=off
  wires:
  Xe/1 -> Demux1/1
  Constant3/1 -> Sum/2
  Demux1/3 -> Sum/1
  Demux1/2 -> Terminator4/1
  Demux1/1 -> Terminator1/1
  Clock/1 -> " 1"/2, " 2"/2
  Constant2/1 -> " 2"/3, " 1"/3
  Gain/1 -> Saturation1/1
  " 1"/1 -> ThetaRef/1, To Workspace1/1
  Constant4/1 -> " 2"/1
  " 2"/1 -> To Workspace/1, psiREF/1
  Sum/1 -> Gain/1
  Saturation1/1 -> " 1"/1

== system GuiamentoControle/Guiamento e Controle/Guiamento Terminal ==
  TetaAD : Inport
  OmegaY : Inport  Port=2
  PsiAD : Inport  Port=3
  OmegaZ : Inport  Port=4
  DCM : Inport  Port=5
  Rastreio : Inport  Port=6
  |Vm| : Inport  Port=7
  Add : Sum  Inputs=|++
  Add1 : Sum  Inputs=|++
  Compensação Gravidade : Subsystem
  Demux : Demux  Outputs=3
  Ganho Prop : Gain  Gain=-D.KProp
  Ganho Prop1 : Gain  Gain=D.KProp
  Multiply : Product  Inputs=**/
  Multiply1 : Product  Inputs=**/
  Product1 : Product  Inputs=**  RndMeth=Zero
  Product2 : Product  Inputs=**  RndMeth=Zero
  Terminator : Terminator
  To Workspace : ToWorkspace  VariableName=CompGrav  SaveFormat=Timeseries  SampleTime=-1
  To Workspace1 : ToWorkspace  VariableName=AcelZNP  SaveFormat=Timeseries  SampleTime=-1
  To Workspace2 : ToWorkspace  VariableName=AcelYNP  SaveFormat=Timeseries  SampleTime=-1
  Trigonometric Function1 : Trigonometry  Operator=cos
  Trigonometric Function2 : Trigonometry  Operator=cos
  AcelZCom : Outport  VectorParamsAs1DForOutWhenUnconnected=off
  AcelYCom : Outport  Port=2  VectorParamsAs1DForOutWhenUnconnected=off
  wires:
  TetaAD/1 -> Trigonometric Function2/1
  OmegaY/1 -> Ganho Prop/1
  Ganho Prop/1 -> Multiply/1
  Trigonometric Function2/1 -> Multiply/3
  |Vm|/1 -> Multiply1/2, Multiply/2
  Add/1 -> AcelZCom/1
  Trigonometric Function1/1 -> Multiply1/3
  Add1/1 -> AcelYCom/1
  PsiAD/1 -> Trigonometric Function1/1
  OmegaZ/1 -> Ganho Prop1/1
  Ganho Prop1/1 -> Multiply1/1
  Demux/1 -> Terminator/1
  Product2/1 -> Add/1
  Product1/1 -> Add1/1
  Demux/2 -> Add1/2
  Demux/3 -> Add/2
  DCM/1 -> Compensação Gravidade/1(DCM)
  Compensação Gravidade/1(g_b) -> To Workspace/1, Demux/1
  Multiply/1 -> Product2/1, To Workspace1/1
  Multiply1/1 -> Product1/1, To Workspace2/1
  Rastreio/1 -> Product1/2, Product2/2

== system GuiamentoControle/Verifca Fim/Bingo ==
  Rtm : Inport
  Compare To Constant : simulink/Logic and Bit Operations/Compare To Constant  relop=<=  const=D.REspoleta  OutDataTypeStr=boolean  ZeroCross=off
  Sqrt : Sqrt
  Stop Simulation1 : Stop
  To Workspace : ToWorkspace  VariableName=RMiss  SaveFormat=Timeseries  SampleTime=-1
  To Workspace8 : ToWorkspace  VariableName=Bingo  SampleTime=-1
  dot : aerolibasang/Incidence, Sideslip, & Airspeed/dot  SystemSampleTime=-1
      settings: SourceProductName=Aerospace Blockset
  wires:
  Rtm/1 -> dot/1
  dot/1 -> Sqrt/1
  Compare To Constant/1 -> To Workspace8/1, Stop Simulation1/1
  Sqrt/1 -> To Workspace/1, Compare To Constant/1

== system GuiamentoControle/Verifca Fim/Impacto com solo ==
  Rtm : Inport
  Compare To Constant : simulink/Logic and Bit Operations/Compare To Constant  relop=>  const=0  OutDataTypeStr=boolean  ZeroCross=off
  Demux : Demux  Outputs=3
  Stop Simulation1 : Stop
  Terminator : Terminator
  Terminator1 : Terminator
  To Workspace8 : ToWorkspace  VariableName=ImpactoSolo  SampleTime=-1
  wires:
  Rtm/1 -> Demux/1
  Compare To Constant/1 -> To Workspace8/1, Stop Simulation1/1
  Demux/3 -> Compare To Constant/1
  Demux/1 -> Terminator/1
  Demux/2 -> Terminator1/1

== system GuiamentoControle/Verifca Fim/Parada: Fuga do alvo ==
  Rtm : Inport
  Vtm : Inport  Port=2
  t : Inport  Port=3
  Add : Sum  Inputs=+-
  Compare To Zero : simulink/Logic and Bit Operations/Compare To Zero  relop=>  OutDataTypeStr=boolean  ZeroCross=off
  Compare To Zero1 : simulink/Logic and Bit Operations/Compare To Zero  relop=>  OutDataTypeStr=boolean  ZeroCross=off
  Constant : Constant  Value=D.TqB
  Dot Product : DotProduct  OutDataTypeStr=Inherit: Inherit via internal rule
  Logical Operator : Logic  AllPortsSameDT=off  OutDataTypeStr=boolean
  Stop Simulation : Stop
  To Workspace10 : ToWorkspace  VariableName=Stop_FugaAlvo  SampleTime=-1
  wires:
  Rtm/1 -> Dot Product/1
  Dot Product/1 -> Compare To Zero/1
  Compare To Zero/1 -> Logical Operator/1
  Logical Operator/1 -> To Workspace10/1, Stop Simulation/1
  t/1 -> Add/1
  Add/1 -> Compare To Zero1/1
  Compare To Zero1/1 -> Logical Operator/2
  Constant/1 -> Add/2
  Vtm/1 -> Dot Product/2

== system GuiamentoControle/Verifca Fim/Parada: V < VMin ==
  V : Inport
  t : Inport  Port=2
  Compare To Constant : simulink/Logic and Bit Operations/Compare To Constant  relop=<=  const=D.VMin  OutDataTypeStr=boolean
  Compare To Constant1 : simulink/Logic and Bit Operations/Compare To Constant  relop=>=  const=D.TqB  OutDataTypeStr=boolean
  Logical Operator1 : Logic  AllPortsSameDT=off  OutDataTypeStr=boolean
  Sqrt : Sqrt
  Stop Simulation2 : Stop
  To Workspace9 : ToWorkspace  VariableName=Stop_VMin  SampleTime=-1
  dot : aerolibasang/Incidence, Sideslip, & Airspeed/dot  SystemSampleTime=-1
      settings: SourceProductName=Aerospace Blockset
  wires:
  Compare To Constant1/1 -> Logical Operator1/2
  Compare To Constant/1 -> Logical Operator1/1
  Logical Operator1/1 -> To Workspace9/1, Stop Simulation2/1
  t/1 -> Compare To Constant1/1
  dot/1 -> Sqrt/1
  V/1 -> dot/1
  Sqrt/1 -> Compare To Constant/1

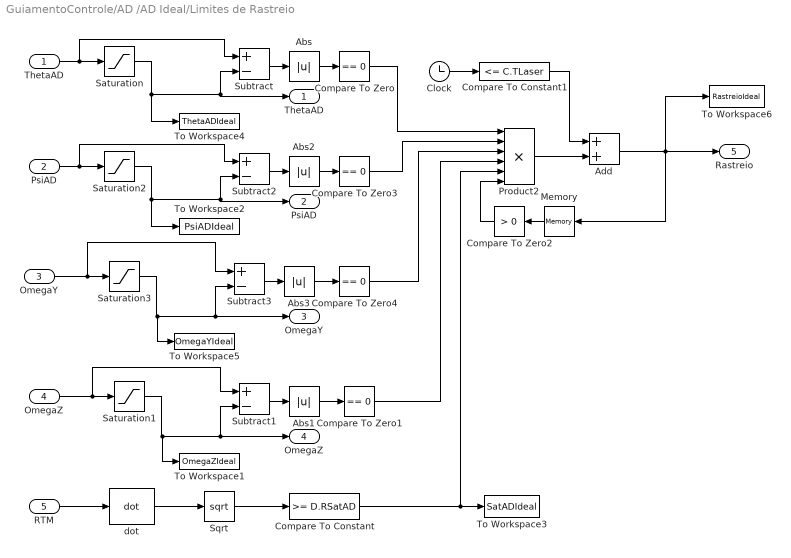
== system GuiamentoControle/AD /AD Ideal/Limites de Rastreio  ==
  ThetaAD : Inport
  PsiAD : Inport  Port=2
  OmegaY : Inport  Port=3
  OmegaZ : Inport  Port=4
  RTM : Inport  Port=5
  Abs{,1..3} (4 alike) : Abs  SaturateOnIntegerOverflow=off
  Add : Sum
  Clock : Clock
  Compare To Constant : simulink/Logic and Bit Operations/Compare To Constant  relop=>=  const=D.RSatAD  OutDataTypeStr=boolean
  Compare To Constant1 : simulink/Logic and Bit Operations/Compare To Constant  relop=<=  const=C.TLaser  OutDataTypeStr=boolean  ZeroCross=off
  Compare To Zero{,1,3..4} (4 alike) : simulink/Logic and Bit Operations/Compare To Zero  relop===  OutDataTypeStr=boolean
  Compare To Zero2 : simulink/Logic and Bit Operations/Compare To Zero  relop=>  OutDataTypeStr=boolean
  Memory : Memory  InitialCondition=1
  Product2 : Product  Inputs=******  RndMeth=Zero
  Saturation : Saturate  UpperLimit=D.ThetaADmax  LowerLimit=-D.ThetaADmax
  Saturation1 : Saturate  UpperLimit=D.OmegaADmax  LowerLimit=-D.OmegaADmax
  Saturation2 : Saturate  UpperLimit=D.ThetaADmax  LowerLimit=-D.ThetaADmax
  Saturation3 : Saturate  UpperLimit=D.OmegaADmax  LowerLimit=-D.OmegaADmax
  Sqrt : Sqrt
  Subtract{,1..3} (4 alike) : Sum  Inputs=+-
  To Workspace1 : ToWorkspace  VariableName=OmegaZIdeal  SaveFormat=Timeseries  SampleTime=-1
  To Workspace2 : ToWorkspace  VariableName=PsiADIdeal  SaveFormat=Timeseries  SampleTime=-1
  To Workspace3 : ToWorkspace  VariableName=SatADIdeal  SaveFormat=Timeseries  SampleTime=-1
  To Workspace4 : ToWorkspace  VariableName=ThetaADIdeal  SaveFormat=Timeseries  SampleTime=-1
  To Workspace5 : ToWorkspace  VariableName=OmegaYIdeal  SaveFormat=Timeseries  SampleTime=-1
  To Workspace6 : ToWorkspace  VariableName=RastreioIdeal  SaveFormat=Timeseries  SampleTime=-1
  dot : aerolibasang/Incidence, Sideslip, & Airspeed/dot  SystemSampleTime=-1  VariantActivationTime=update diagram  AllowFlexibleInterface=on  Latency=0  AutoFrameSizeCalculation=off
  "ThetaAD " : Outport  VectorParamsAs1DForOutWhenUnconnected=off
  "PsiAD " : Outport  Port=2  VectorParamsAs1DForOutWhenUnconnected=off
  "OmegaY " : Outport  Port=3  VectorParamsAs1DForOutWhenUnconnected=off
  "OmegaZ " : Outport  Port=4  VectorParamsAs1DForOutWhenUnconnected=off
  Rastreio : Outport  Port=5  VectorParamsAs1DForOutWhenUnconnected=off
  wires:
  ThetaAD/1 -> Saturation/1, Subtract/1
  Abs/1 -> Compare To Zero/1
  Abs1/1 -> Compare To Zero1/1
  Saturation/1 -> To Workspace4/1, "ThetaAD "/1, Subtract/2
  OmegaZ/1 -> Subtract1/1, Saturation1/1
  Compare To Zero/1 -> Product2/1
  Subtract/1 -> Abs/1
  Memory/1 -> Compare To Zero2/1
  Subtract1/1 -> Abs1/1
  Saturation1/1 -> To Workspace1/1, "OmegaZ "/1, Subtract1/2
  Compare To Constant/1 -> To Workspace3/1, Product2/5
  Sqrt/1 -> Compare To Constant/1
  RTM/1 -> dot/1
  dot/1 -> Sqrt/1
  Compare To Zero2/1 -> Product2/6
  Subtract2/1 -> Abs2/1
  Saturation2/1 -> To Workspace2/1, Subtract2/2, "PsiAD "/1
  PsiAD/1 -> Saturation2/1, Subtract2/1
  Abs2/1 -> Compare To Zero3/1
  Compare To Zero3/1 -> Product2/2
  Subtract3/1 -> Abs3/1
  Abs3/1 -> Compare To Zero4/1
  Saturation3/1 -> To Workspace5/1, Subtract3/2, "OmegaY "/1
  OmegaY/1 -> Subtract3/1, Saturation3/1
  Compare To Zero4/1 -> Product2/3
  Compare To Zero1/1 -> Product2/4
  Clock/1 -> Compare To Constant1/1
  Product2/1 -> Add/2
  Compare To Constant1/1 -> Add/1
  Add/1 -> Memory/1, To Workspace6/1, Rastreio/1

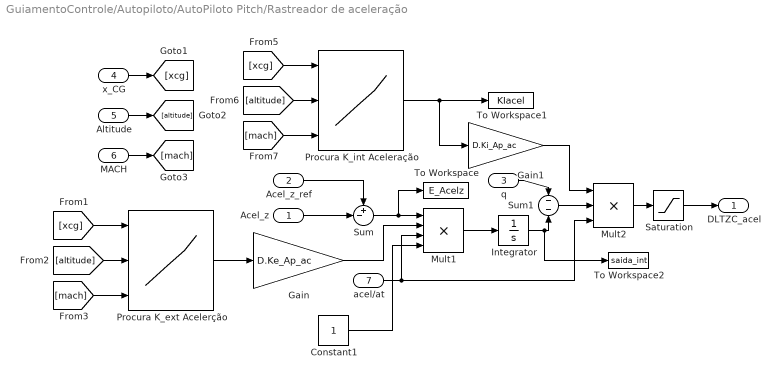
== system GuiamentoControle/Autopiloto/AutoPiloto Pitch/Rastreador de aceleração ==
  Acel_z : Inport
  Acel_z_ref : Inport  Port=2
  q : Inport  Port=3
  x_CG : Inport  Port=4
  Altitude : Inport  Port=5
  MACH : Inport  Port=6
  acel/at : Inport  Port=7
  Constant1 : Constant
  Gain : Gain  Gain=D.Ke_Ap_ac
  Gain1 : Gain  Gain=D.Ki_Ap_ac
  Integrator : Integrator  LimitOutput=on  UpperSaturationLimit=D.sat_integAP  LowerSaturationLimit=-D.sat_integAP
  Mult1 : Product  Inputs=****
  Mult2 : Product  Inputs=***
  Procura K_ext Acelerção : Lookup_n-D  NumberOfTableDimensions=3  BreakpointsForDimension1=vet_x_CG  BreakpointsForDimension2=vet_altitude  BreakpointsForDimension3=vet_Mach  Table=T_acel_k_ext  ExtrapMethod=Clip  RndMeth=Simplest
      settings: InputPortMap=u0,u1,u2
  Procura K_int Aceleração : Lookup_n-D  NumberOfTableDimensions=3  BreakpointsForDimension1=vet_x_CG  BreakpointsForDimension2=vet_altitude  BreakpointsForDimension3=vet_Mach  Table=T_acel_k_int  ExtrapMethod=Clip  RndMeth=Simplest
      settings: InputPortMap=u0,u1,u2
  Saturation : Saturate  UpperLimit=D.Dlt_max - D.Dlt_max_roll  LowerLimit=-D.Dlt_max + D.Dlt_max_roll
  Sum : Sum  Inputs=+-|
  Sum1 : Sum  Inputs=--
  To Workspace : ToWorkspace  VariableName=E_Acelz  SaveFormat=Timeseries  SampleTime=-1
  To Workspace1 : ToWorkspace  VariableName=KIacel  SaveFormat=Timeseries  SampleTime=-1
  To Workspace2 : ToWorkspace  VariableName=saida_int  SaveFormat=Timeseries  SampleTime=-1
  DLTZC_acel : Outport  VectorParamsAs1DForOutWhenUnconnected=off
  wires:
  Procura K_ext Acelerção/1 -> Gain/1
  Sum/1 -> To Workspace/1, Mult1/1
  Acel_z_ref/1 -> Sum/1
  Acel_z/1 -> Sum/2
  Mult1/1 -> Integrator/1
  q/1 -> Sum1/1
  x_CG/1 -> [xcg]
  Altitude/1 -> [altitude]
  MACH/1 -> [mach]
  [altitude] -> Procura K_int Aceleração/2
  [xcg] -> Procura K_int Aceleração/1
  [mach] -> Procura K_int Aceleração/3
  [xcg] -> Procura K_ext Acelerção/1
  [altitude] -> Procura K_ext Acelerção/2
  [mach] -> Procura K_ext Acelerção/3
  Procura K_int Aceleração/1 -> Gain1/1, To Workspace1/1
  Mult2/1 -> Saturation/1
  Gain1/1 -> Mult2/1
  Sum1/1 -> Mult2/2
  Gain/1 -> Mult1/2
  acel/at/1 -> Mult2/3, Mult1/3
  Integrator/1 -> To Workspace2/1, Sum1/2
  Saturation/1 -> DLTZC_acel/1
  Constant1/1 -> Mult1/4

== system GuiamentoControle/Autopiloto/AutoPiloto Pitch/Rastreador de atitude ==
  Theta : Inport
  Theta_ref : Inport  Port=2
  q : Inport  Port=3
  x_CG : Inport  Port=4
  Altitude : Inport  Port=5
  MACH : Inport  Port=6
  Gain : Gain  Gain=D.Ke_Ap_at
  Gain1 : Gain  Gain=D.Ki_Ap_at
  Mult : Product  Inputs=**
  Mult1 : Product  Inputs=**
  Procura K_ext Atitude : Lookup_n-D  NumberOfTableDimensions=3  BreakpointsForDimension1=vet_x_CG  BreakpointsForDimension2=vet_altitude  BreakpointsForDimension3=vet_Mach  Table=T_at_k_ext  ExtrapMethod=Clip  RndMeth=Simplest
      settings: InputPortMap=u0,u1,u2
  Procura K_int Atitude : Lookup_n-D  NumberOfTableDimensions=3  BreakpointsForDimension1=vet_x_CG  BreakpointsForDimension2=vet_altitude  BreakpointsForDimension3=vet_Mach  Table=T_at_k_int  ExtrapMethod=Clip  RndMeth=Simplest
      settings: InputPortMap=u0,u1,u2
  Saturation : Saturate  UpperLimit=D.Dlt_max - D.Dlt_max_roll  LowerLimit=-D.Dlt_max + D.Dlt_max_roll
  Sum : Sum  Inputs=|+-
  Sum1 : Sum  Inputs=|+-
  DLTZC_atitude : Outport  VectorParamsAs1DForOutWhenUnconnected=off
  wires:
  Procura K_ext Atitude/1 -> Gain/1
  Procura K_int Atitude/1 -> Gain1/1
  Gain1/1 -> Mult/1
  x_CG/1 -> [xcg]
  Altitude/1 -> [altitude]
  MACH/1 -> [mach]
  [xcg] -> Procura K_int Atitude/1
  [altitude] -> Procura K_int Atitude/2
  [mach] -> Procura K_int Atitude/3
  [mach] -> Procura K_ext Atitude/3
  [altitude] -> Procura K_ext Atitude/2
  [xcg] -> Procura K_ext Atitude/1
  Saturation/1 -> DLTZC_atitude/1
  Sum1/1 -> Mult/2
  Mult/1 -> Saturation/1
  q/1 -> Sum1/2
  Mult1/1 -> Sum1/1
  Theta/1 -> Sum/2
  Theta_ref/1 -> Sum/1
  Gain/1 -> Mult1/1
  Sum/1 -> Mult1/2

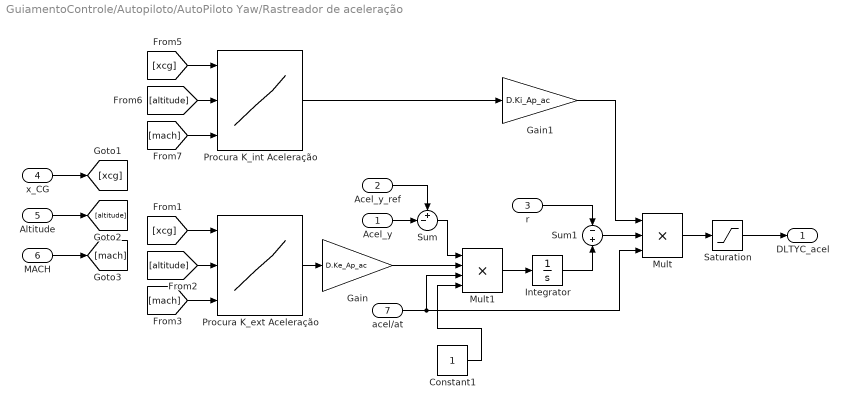
== system GuiamentoControle/Autopiloto/AutoPiloto Yaw/Rastreador de aceleração ==
  Acel_y : Inport
  Acel_y_ref : Inport  Port=2
  r : Inport  Port=3
  x_CG : Inport  Port=4
  Altitude : Inport  Port=5
  MACH : Inport  Port=6
  acel/at : Inport  Port=7
  Constant1 : Constant
  Gain : Gain  Gain=D.Ke_Ap_ac
  Gain1 : Gain  Gain=D.Ki_Ap_ac
  Integrator : Integrator  LimitOutput=on  UpperSaturationLimit=D.sat_integAP  LowerSaturationLimit=-D.sat_integAP
  Mult : Product  Inputs=***
  Mult1 : Product  Inputs=****
  Procura K_ext Aceleração : Lookup_n-D  NumberOfTableDimensions=3  BreakpointsForDimension1=vet_x_CG  BreakpointsForDimension2=vet_altitude  BreakpointsForDimension3=vet_Mach  Table=T_acel_k_ext  ExtrapMethod=Clip  RndMeth=Simplest
      settings: InputPortMap=u0,u1,u2
  Procura K_int Aceleração : Lookup_n-D  NumberOfTableDimensions=3  BreakpointsForDimension1=vet_x_CG  BreakpointsForDimension2=vet_altitude  BreakpointsForDimension3=vet_Mach  Table=T_acel_k_int  ExtrapMethod=Clip  RndMeth=Simplest
      settings: InputPortMap=u0,u1,u2
  Saturation : Saturate  UpperLimit=D.Dlt_max - D.Dlt_max_roll  LowerLimit=-D.Dlt_max + D.Dlt_max_roll
  Sum : Sum  Inputs=+-|
  Sum1 : Sum  Inputs=-+
  DLTYC_acel : Outport  VectorParamsAs1DForOutWhenUnconnected=off
  wires:
  Mult1/1 -> Integrator/1
  Procura K_ext Aceleração/1 -> Gain/1
  Sum/1 -> Mult1/1
  Gain/1 -> Mult1/2
  Procura K_int Aceleração/1 -> Gain1/1
  x_CG/1 -> [xcg]
  Altitude/1 -> [altitude]
  MACH/1 -> [mach]
  [xcg] -> Procura K_int Aceleração/1
  [altitude] -> Procura K_int Aceleração/2
  [mach] -> Procura K_int Aceleração/3
  [xcg] -> Procura K_ext Aceleração/1
  [altitude] -> Procura K_ext Aceleração/2
  [mach] -> Procura K_ext Aceleração/3
  Acel_y_ref/1 -> Sum/1
  Acel_y/1 -> Sum/2
  acel/at/1 -> Mult/3, Mult1/3
  Saturation/1 -> DLTYC_acel/1
  r/1 -> Sum1/1
  Mult/1 -> Saturation/1
  Integrator/1 -> Sum1/2
  Gain1/1 -> Mult/1
  Sum1/1 -> Mult/2
  Constant1/1 -> Mult1/4

== system GuiamentoControle/Autopiloto/AutoPiloto Yaw/Rastreador de atitude ==
  r : Inport
  x_CG : Inport  Port=2
  Altitude : Inport  Port=3
  MACH : Inport  Port=4
  Psi : Inport  Port=5
  Psi_ref : Inport  Port=6
  Gain : Gain  Gain=D.Ke_Ap_at
  Gain1 : Gain  Gain=D.Ki_Ap_at
  Mult : Product  Inputs=**
  Mult1 : Product  Inputs=**
  Procura K_ext Atitude : Lookup_n-D  NumberOfTableDimensions=3  BreakpointsForDimension1=vet_x_CG  BreakpointsForDimension2=vet_altitude  BreakpointsForDimension3=vet_Mach  Table=T_at_k_ext  ExtrapMethod=Clip  RndMeth=Simplest
      settings: InputPortMap=u0,u1,u2
  Procura K_int Atitude : Lookup_n-D  NumberOfTableDimensions=3  BreakpointsForDimension1=vet_x_CG  BreakpointsForDimension2=vet_altitude  BreakpointsForDimension3=vet_Mach  Table=T_at_k_int  ExtrapMethod=Clip  RndMeth=Simplest
      settings: InputPortMap=u0,u1,u2
  Saturation : Saturate  UpperLimit=D.Dlt_max - D.Dlt_max_roll  LowerLimit=-D.Dlt_max + D.Dlt_max_roll
  Sum : Sum  Inputs=|+-
  Sum1 : Sum  Inputs=-+
  DLTYC_atitude : Outport  VectorParamsAs1DForOutWhenUnconnected=off
  wires:
  Mult1/1 -> Sum1/2
  Procura K_ext Atitude/1 -> Gain/1
  Procura K_int Atitude/1 -> Gain1/1
  Gain1/1 -> Mult/1
  r/1 -> Sum1/1
  x_CG/1 -> [xcg]
  Altitude/1 -> [altitude]
  MACH/1 -> [mach]
  [xcg] -> Procura K_int Atitude/1
  [altitude] -> Procura K_int Atitude/2
  [mach] -> Procura K_int Atitude/3
  [xcg] -> Procura K_ext Atitude/1
  [altitude] -> Procura K_ext Atitude/2
  [mach] -> Procura K_ext Atitude/3
  Saturation/1 -> DLTYC_atitude/1
  Sum1/1 -> Mult/2
  Mult/1 -> Saturation/1
  Psi/1 -> Sum/2
  Psi_ref/1 -> Sum/1
  Gain/1 -> Mult1/1
  Sum/1 -> Mult1/2

== system GuiamentoControle/Dinâmica 6DOF/Aerodinâmica 2D/Calcula Momentos no CG ==
  Forces : Inport
  CRM : Inport  Port=2
  CG : Inport  Port=3
  Moments CRM : Inport  Port=4
  3x3 Cross Product : sharedutil/3x3 Cross Product  aMode=aMode
  Sum : Sum  Inputs=|+-  SaturateOnIntegerOverflow=on
  Sum1 : Sum  Inputs=|++  SaturateOnIntegerOverflow=on
  To Workspace : ToWorkspace  VariableName=Delta_CG  SaveFormat=Timeseries  SampleTime=-1
  Moments CG : Outport  VectorParamsAs1DForOutWhenUnconnected=off
  wires:
  CRM/1 -> Sum/1
  CG/1 -> Sum/2
  Sum/1 -> 3x3 Cross Product/1, To Workspace/1
  Forces/1 -> 3x3 Cross Product/2
  Moments CRM/1 -> Sum1/2
  Sum1/1 -> Moments CG/1
  3x3 Cross Product/1 -> Sum1/1
